simulink model "pendule_inverse_force"  (R2016a)
settings: Solver=VariableStepAuto  StartTime=0.0  StopTime=12.6874796984388  RelTol=1e-4
undefined symbols (not defined in the file): DiscIntNeverNeededParam
libraries: simulink x1
settings Model: Creator=tmeunier  LastModifiedBy=tmeunier

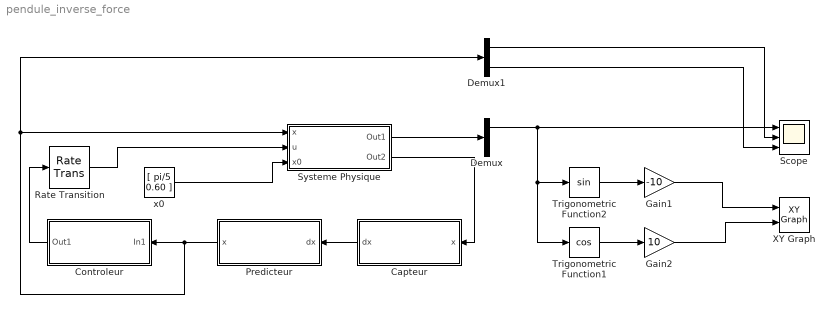
== system pendule_inverse_force ==
  Capteur : Subsystem
  Controleur : Subsystem
  Demux : Demux  Outputs=2
  Demux1 : Demux  Outputs=2
  Gain1 : Gain  Gain=-10
  Gain2 : Gain  Gain=10
  Predicteur : Subsystem
  Rate Transition : RateTransition
  Scope : Scope  NumInputPorts=3
  Systeme Physique : Subsystem
  Trigonometric Function1 : Trigonometry  Operator=cos
  Trigonometric Function2 : Trigonometry
  XY Graph : simulink/Sinks/XY Graph  xmin=-10  xmax=10  ymin=-10  ymax=10  st=-1
  x0 : Constant  Value=[ pi/5 0.60 ]
  wires:
  Gain1/1 -> XY Graph/1
  Trigonometric Function2/1 -> Gain1/1
  Trigonometric Function1/1 -> Gain2/1
  Gain2/1 -> XY Graph/2
  Systeme Physique/1(Out1) -> Demux/1
  Demux/1 -> Trigonometric Function1/1, Trigonometric Function2/1, Scope/1
  Demux1/2 -> Scope/3
  Demux1/1 -> Scope/2
  x0/1 -> Systeme Physique/3(x0)
  Capteur/1(dx) -> Predicteur/1(dx)
  Systeme Physique/2(Out2) -> Capteur/1(x)
  Predicteur/1(x) -> Demux1/1, Systeme Physique/1(x), Controleur/1(In1)
  Controleur/1(Out1) -> Rate Transition/1
  Rate Transition/1 -> Systeme Physique/2(u)

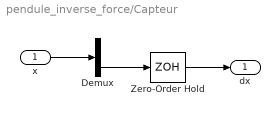
== system pendule_inverse_force/Capteur ==
  x : Inport
  Demux : Demux  Outputs=2
  Zero-Order Hold : ZeroOrderHold  SampleTime=25*12.61/500
  dx : Outport
  wires:
  x/1 -> Demux/1
  Zero-Order Hold/1 -> dx/1
  Demux/2 -> Zero-Order Hold/1

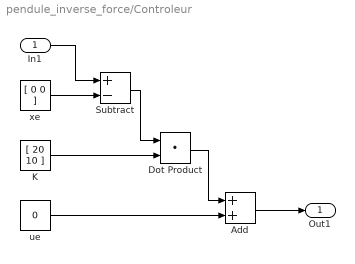
== system pendule_inverse_force/Controleur ==
  In1 : Inport
  Add : Sum
  Dot Product : DotProduct  InputSameDT=on  OutDataTypeStr=Inherit: Inherit via internal rule
  K : Constant  Value=[ 20 10 ]
  Subtract : Sum  Inputs=+-
  ue : Constant  Value=0
  xe : Constant  Value=[ 0 0 ]
  Out1 : Outport
  wires:
  xe/1 -> Subtract/2
  In1/1 -> Subtract/1
  Subtract/1 -> Dot Product/1
  K/1 -> Dot Product/2
  Dot Product/1 -> Add/1
  ue/1 -> Add/2
  Add/1 -> Out1/1

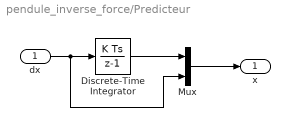
== system pendule_inverse_force/Predicteur ==
  dx : Inport
  Discrete-Time Integrator : DiscreteIntegrator  InitialConditionSetting=State (most efficient)  SampleTime=25*12.61/500  ICPrevOutput=DiscIntNeverNeededParam  ICPrevScaledInput=DiscIntNeverNeededParam
  Mux : Mux  Inputs=2
  x : Outport
  wires:
  dx/1 -> Mux/2, Discrete-Time Integrator/1
  Discrete-Time Integrator/1 -> Mux/1
  Mux/1 -> x/1

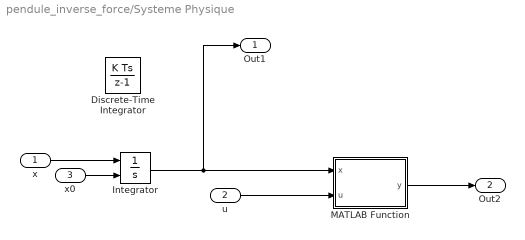
== system pendule_inverse_force/Systeme Physique ==
  x : Inport
  u : Inport  Port=2
  x0 : Inport  Port=3
  Discrete-Time Integrator : DiscreteIntegrator  InitialConditionSetting=State (most efficient)  ICPrevOutput=DiscIntNeverNeededParam  ICPrevScaledInput=DiscIntNeverNeededParam
  Integrator : Integrator  InitialConditionSource=external  InitialCondition=[ pi/5 0.60 ]
  MATLAB Function : MATLAB Function  TreatAsAtomicUnit=on
  Out1 : Outport
  Out2 : Outport  Port=2
  wires:
  u/1 -> MATLAB Function/2(u)
  Integrator/1 -> Out1/1, MATLAB Function/1(x)
  x/1 -> Integrator/1
  MATLAB Function/1(y) -> Out2/1
  x0/1 -> Integrator/2

== matlab function pendule_inverse_force/Systeme Physique/MATLAB Function ==
  data: x input; u input; y output
function y = f(x, u)

%% Constants
g = 9.81;
l = 10;

%% Controle
dx = zeros(1, 2);

dx(1) = x(2);
dx(2) = g/l*sin(x(1)) - u*cos(x(1))/l;
y = [ dx(2) dx(1) ];
